simulink model "sedemo_event_translation_stateflow"  (Simulink 7.5)
settings: Solver=VariableStepDiscrete  StartTime=0.0  StopTime=20  MaxStep=0.2  RelTol=1e-3
libraries: simeventssink1 x3, simeventsgenerators1 x2, simeventsqueue1 x1, simeventssignalmanage1 x1, simeventstranslate1 x1, simeventsserver1 x1
settings Model: Creator=The MathWorks Inc.
settings OptimizationCC: InitFltsAndDblsToZero=on  EfficientMapNaN2IntZero=off
settings DebuggingCC: StrictBusMsg=Warning
settings SimEventsCC: propDiagAttribOutput=1  propDiagFcnCallOutput=1  propDiagStatOutput=0

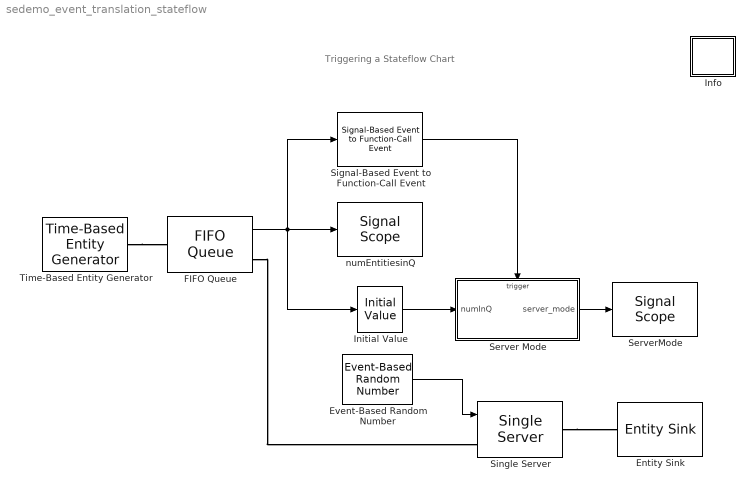
== system sedemo_event_translation_stateflow ==
  note: Triggering a Stateflow Chart
  Entity Sink : simeventssink1/Entity Sink  Priority=1  SystemSampleTime=-1  AvailableForArrivals=on  StatNumberArrived=Off
  Event-Based Random Number : simeventsgenerators1/Signal Generators/Event-Based Random Number  SystemSampleTime=-1  distribution=Exponential  meanExp=1.5  minUnif=1  maxUnif=1  pOneBern=0.25  pSuccessBino=0.5  numTrialBino=1  meanNorm=0  stdNorm=1  minTri=1  maxTri=3  modeTri=2  thresholdLogn=0  scaleLogn=1  shapeLogn=1  pSuccessGeo=0.5  meanPoiss=1  thresholdLogl=0  scaleLogl=1  thresholdGam=0  scaleGam=1  shapeGam=1  minBeta=0  maxBeta=1  shape1Beta=1  shape2Beta=1  minUnid=0  maxUnid=1  numValueUnid=2  thresholdWbl=0  scaleWbl=1  shapeWbl=1  valueVecCont=[0 1]  cdfVecCont=[0 1]  valueVecDisc=[0 1]  probVecDisc=[0.5 0.5]  seed=154647  IsProcessed=on  isConnected=1
  FIFO Queue : simeventsqueue1/FIFO Queue  Priority=1  SystemSampleTime=-1  Capacity=25  EnableTOPort=off  StatNumberDeparted=Off  StatNumberInBlock=On  StatPendingEntity=Off  StatAverageWait=Off  StatAverageQueueLength=Off  StatNumberTimedout=Off
  Info : Subsystem
      settings: OpenFcn=simeventsdemohelp('sedemo_event_translation');
      mask Type: Info About This Model
      mask Help: evalc(['simeventsdemohelp(''sedemo_event_translation'');']);
      mask Display: disp('Info')
  Initial Value : simeventssignalmanage1/Initial Value  InitialValue=1
  Server Mode : Stateflow chart  TreatAsAtomicUnit=on
      settings: PropExecContextOutsideSubsystem=on
  ServerMode : simeventssink1/Signal Scope  Priority=1  SystemSampleTime=-1  PlotType=Stair  InputType=Signal  NumInputs=1  AttributeNameY=Count  XInputOptionSignal=Event time  XInputOptionEntity=Event time  AttributeNameX=Count  EnableEntityOutport=on  XMin=1.69504025250588  XMax=20.4586541286158  XLimitExceededOption=Stretch axis limits  YLimitExceededOption=Stretch axis limits  AxisGrid=on  AxisLegend=off  LineDisables=""  LineColors=b  LineStyles=-  LineMarkers=.  OpenScopeAtSimStart=on  Title=Server Mode  YLabel=""  XLabel=Time  FigurePosition=[287 57 256 192]  AxisZoom=off  DataStoreOption=Limited  DataPointsLimit=10000  StatNumberArrived=Off  ShowCountPlotted=off  ShowToolbar=on
      settings: YMin=-0.00356032002678863  YMax=2.62744183433855
  Signal-Based Event to Function-Call Event : simeventstranslate1/Signal-Based Event to Function-Call Event  Priority=1  SystemSampleTime=-1  GenerateFunctionCallUpon=Change in signal from port vc  SignalEdgeOption=Either  EnableE1Port=off  EnableF2Port=off  EnableE2Port=off  SpecifyEventPriority=off  PriorityFunctionCall=200  FunctionCallDelayFrom=Dialog  DelayFunctionCall=0  StatNumberF1Calls=Off  StatNumberF2Calls=Off  MaskBlockType=none
  Single Server : simeventsserver1/Single Server  Priority=1  SystemSampleTime=-1  ServiceTimeFrom=Signal port t  ServiceTime=5  AttributeName=ServiceTime  PriorityServiceCompletion=500  PermitPreemption=off  SortingAttributeName=PriorityAttributeName  SortingDirection=Ascending  WriteToAttribute=off  ResidualAttributeName=ResidualServiceTime  CreateAttribute=on  EnableTOPort=off  StatNumberDeparted=Off  StatNumberInBlock=Off  StatNumberPreempted=Off  StatPendingEntity=Off  StatAverageWait=Off  StatUtilization=Off  StatNumberTimedout=Off
  Time-Based Entity Generator : simeventsgenerators1/Entity Generators/Time-Based Entity Generator  Priority=1  DialogController=des_ddg_create  DialogControllerArgs=DataTag6  SystemSampleTime=-1  GenerateEntitiesUpon=Intergeneration time from dialog  Distribution=Uniform  Minimum=1  Maximum=1.2  Mean=1.2  InitialSeed=45983  Period=1  PriorityEntityGeneration=300  GenerateEntityAtSimulationStart=on  ResponseWhenBlocked=Pause generation  ResponseWhenUnblocked=Immediate restart  EntityType=Blank  StatNumberDeparted=Off  StatPendingEntity=Off  StatAverageIntergenerationTime=Off
  numEntitiesinQ : simeventssink1/Signal Scope  Priority=1  SystemSampleTime=-1  PlotType=Stair  InputType=Signal  NumInputs=1  AttributeNameY=Count  XInputOptionSignal=Event time  XInputOptionEntity=Event time  AttributeNameX=Count  EnableEntityOutport=on  XMin=-0.0527853709114936  XMax=20.2384767650109  XLimitExceededOption=Stretch axis limits  YLimitExceededOption=Stretch axis limits  AxisGrid=on  AxisLegend=off  LineDisables=""  LineColors=b  LineStyles=-  LineMarkers=.  OpenScopeAtSimStart=on  Title=Number of Entities in FIFO Queue  YLabel=""  XLabel=Time  FigurePosition=[24 58 256 192]  AxisZoom=off  DataStoreOption=Limited  DataPointsLimit=10000  StatNumberArrived=Off  ShowCountPlotted=off  ShowToolbar=on
      settings: YMin=-0.0309056705186777  YMax=5.23649556570814
  wires:
  FIFO Queue/1 -> numEntitiesinQ/1, Initial Value/1, Signal-Based Event to Function-Call Event/1
  Signal-Based Event to Function-Call Event/1 -> Server Mode/Trigger
  Server Mode/1(server_mode) -> ServerMode/1
  Initial Value/1 -> Server Mode/1(numInQ)
  Event-Based Random Number/1 -> Single Server/1
  connections:
  Time-Based Entity Generator/RConn1 -- FIFO Queue/LConn1
  FIFO Queue/RConn1 -- Single Server/LConn1
  Single Server/RConn1 -- Entity Sink/LConn1

== system sedemo_event_translation_stateflow/Info ==

== stateflow chart Server Mode ==
  state Up
    en: server_mode=1;
  state Down
    en: server_mode=2;
  Up -> Down : [numInQ<=4]
  Down -> Up : [numInQ>4]
  (default) -> Down
  data: server_mode output double; numInQ input double
  events: event input FUNCTION_CALL_EVENT
